simulink model "InvPendIdent"  (Simulink 8.6)
settings: Solver=ode1  SolverMode=SingleTasking  StartTime=0.0  StopTime=40  FixedStep=0.001  RelTol=1e-3
undefined symbols (not defined in the file): Advantech, magnitude, PCI
libraries: sldrtlib x11, simulink x6
settings Model: Creator=Administrator  LastModifiedBy=demo  SimulationMode=external  ExtModeTrigMode=oneshot  ExtModeTrigDuration=100000
settings DataIOCC: LimitDataPoints=off  SignalLoggingName=sigsOut
settings OptimizationCC: BlockReduction=off  BooleanDataType=off  InitFltsAndDblsToZero=on
settings DebuggingCC: SaveWithParameterizedLinksMsg=none  SignalResolutionControl=TryResolveAllWithWarning  SolverPrmCheckMsg=none  MultiTaskDSMMsg=warning  MultiTaskCondExecSysMsg=none  FcnCallInpInsideContextMsg=UseLocalSettings
settings HardwareCC: ProdBitPerLong=64  ProdBitPerPointer=64  ProdIntDivRoundTo=Zero  ProdEndianess=LittleEndian  ProdWordSize=64  ProdHWDeviceType=Intel->x86-64  TargetBitPerLong=64  TargetBitPerPointer=64  TargetIntDivRoundTo=Zero  TargetEndianess=LittleEndian  TargetWordSize=64  TargetHWDeviceType=Intel->x86-64
settings RTWCC: SystemTargetFile=sldrt.tlc  TemplateMakefile=sldrt.tmf  Description=Simulink Desktop Real-Time  RTWCompilerOptimization=on
settings CodeAppCC: MaxIdLength=95
settings SimulinkDesktopRealTimeCC: TargetPreCompLibLocation=C:\Program Files\MATLAB\R2015b\toolbox\sldrt\lib\win64  TargetLangStandard=C89/C90 (ANSI)  SupportVariableSizeSignals=off

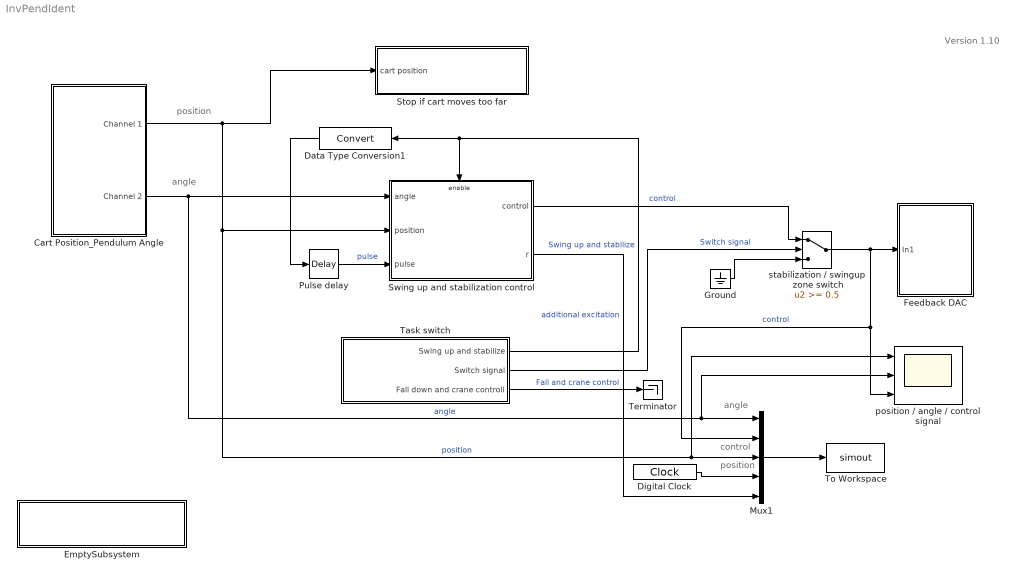
== system InvPendIdent ==
  note: position
  note: angle
  note: Version 1.10
  note: angle
  note: position
  note: control
  Cart Position_Pendulum Angle : Subsystem  mask(Feedback Encoder Block){st=0.001, of1=0, of2=-1024}
      mask prompts: st "Sample Time"; of1 "Channel 1 Offset"; of2 "Channel 2 Offset"
      mask help: Special block to use with the Feedback experiments to read encoder channels using the digital I/O lines
      mask Display:
      | image(imread('bckg.bmp'))
      | disp('PCI1711 \n Lab I/O Board \n\n\n Feedback Encoder')
  Data Type Conversion1 : DataTypeConversion
  Digital Clock : DigitalClock  SampleTime=0.001
  EmptySubsystem : Subsystem
      mask Display:
      | image(imread('FB-inst-blue2.jpg'))
      | disp('\n\nFeedback Instruments Limited')
  Feedback DAC : Subsystem  mask(DAC Unit for Feedback Experiments){st=0.001, ch=1}
      mask prompts: st "Sample Time"; ch "Output Channel"
      mask help:
      | Digital to Analog Output  for Feedback Experiments
      | using Advantech PCI1711  I/O board
      mask Display:
      | image(imread('bckg.bmp'))
      | disp('PCI1711 \n Lab I/O Board \n\n Feedback  DAC')
  Ground : Ground
  Mux1 : Mux  Inputs=5
  Pulse delay : TransportDelay  DelayTime=0.3  FixedBuffer=on
  Stop if cart moves too far : Subsystem
      mask Display:
      | image(imread('bckg.bmp'))
      | disp('Stop if cart moves too far')
  Swing up and stabilization control : Subsystem  TreatAsAtomicUnit=on
      mask Display:
      | image(imread('bckg.bmp'))
      | disp('Swing up \nand stabilization control')
  Task switch : Subsystem
      mask Display:
      | image(imread('bckg.bmp'))
      | disp('Task switch')
  Terminator : Terminator
  To Workspace : ToWorkspace  VariableName=simout  SampleTime=0.001
  position / angle / control signal : Scope  NumInputPorts=3
      mask Display: image(imread('scope.jpg'))
  stabilization / swingup  zone switch : Switch  Threshold=0.5
  wires:
  Cart Position_Pendulum Angle/1(Channel 1) -> Stop if cart moves too far/1(cart position), Swing up and stabilization control/2(position), Mux1/3, position / angle / control signal/1  "position"
  Cart Position_Pendulum Angle/2(Channel 2) -> Swing up and stabilization control/1(angle), Mux1/1, position / angle / control signal/2  "angle"
  stabilization / swingup  zone switch/1 -> Feedback DAC/1(In1), Mux1/2, position / angle / control signal/3  "control"
  Swing up and stabilization control/1(control) -> stabilization / swingup  zone switch/1  "control"
  Pulse delay/1 -> Swing up and stabilization control/3(pulse)  "pulse"
  Data Type Conversion1/1 -> Pulse delay/1
  Task switch/2(Switch signal) -> stabilization / swingup  zone switch/2  "Switch signal"
  Mux1/1 -> To Workspace/1
  Task switch/3(Fall down and crane controll) -> Terminator/1  "Fall and crane control"
  Ground/1 -> stabilization / swingup  zone switch/3
  Task switch/1(Swing up and stabilize) -> Data Type Conversion1/1, Swing up and stabilization control/Enable  "Swing up and stabilize"
  Digital Clock/1 -> Mux1/4
  Swing up and stabilization control/2(r) -> Mux1/5  "additional excitation"

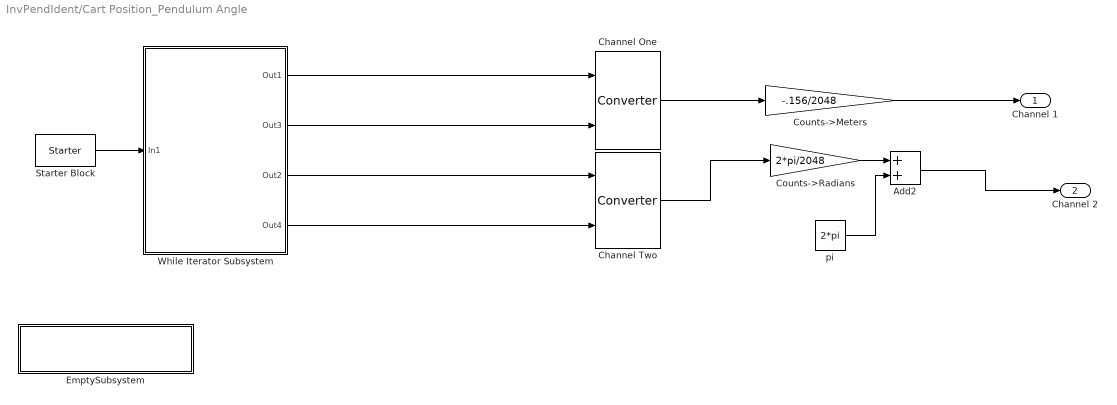
== system InvPendIdent/Cart Position_Pendulum Angle ==
  Add2 : Sum
  Channel One : S-Function  FunctionName=Converter  Parameters=of1,st  SFunctionDeploymentMode=off  EnableBusSupport=off
  Channel Two : S-Function  FunctionName=Converter  Parameters=of2,st  SFunctionDeploymentMode=off  EnableBusSupport=off
  Counts->Meters : Gain  Gain=-.156/2048  SaturateOnIntegerOverflow=on  OutDataTypeStr=Inherit: Same as input  ParamDataTypeStr=Inherit: Same as input
  Counts->Radians : Gain  Gain=2*pi/2048  SaturateOnIntegerOverflow=on  OutDataTypeStr=Inherit: Same as input  ParamDataTypeStr=Inherit: Same as input
  EmptySubsystem : Subsystem
      mask Display:
      | image(imread('FB-inst-blue2.jpg'))
      | disp('\n\nFeedback Instruments Limited')
  Starter Block : S-Function  FunctionName=Starter  Parameters=sample_time  SFunctionDeploymentMode=off  EnableBusSupport=off  mask{sample_time=st}
      mask prompts: sample_time "Sample Time:"
  While Iterator Subsystem : Subsystem  TreatAsAtomicUnit=on
  pi : Constant  Value=2*pi
  Channel 1 : Outport
  Channel 2 : Outport  Port=2
  wires:
  Add2/1 -> Channel 2/1
  Channel Two/1 -> Counts->Radians/1
  pi/1 -> Add2/2
  Counts->Radians/1 -> Add2/1
  Counts->Meters/1 -> Channel 1/1
  Starter Block/1 -> While Iterator Subsystem/1(In1)
  While Iterator Subsystem/1(Out1) -> Channel One/1
  While Iterator Subsystem/2(Out3) -> Channel One/2
  While Iterator Subsystem/3(Out2) -> Channel Two/1
  While Iterator Subsystem/4(Out4) -> Channel Two/2
  Channel One/1 -> Counts->Meters/1

== system InvPendIdent/EmptySubsystem ==

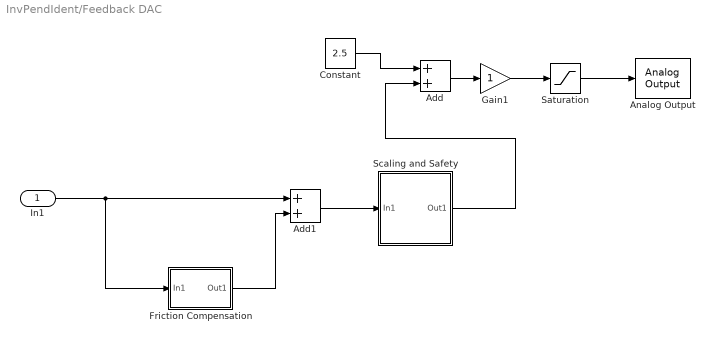
== system InvPendIdent/Feedback DAC ==
  In1 : Inport
  Add : Sum  OutDataTypeStr=Inherit: Same as first input
  Add1 : Sum
  Analog Output : sldrtlib/Analog Output  SampleTime=st  MaxMissedTicks=10  ShowMissedTicks=off  YieldWhenWaiting=off  DrvName=Advantech/PCI-1711  DrvAddress=4294967295  DrvOptions=zeros(1,0)  Channels=ch  RangeMode=1  VoltRange=2  InitialValue=2.5  FinalValue=2.5
      settings: AttributesFormatString=Advantech\nPCI-1711 [auto]
  Constant : Constant  Value=2.5
  Friction Compensation : Subsystem  mask(linear){frictionCompNeg=.1, frictionCompPos=.1}
      mask prompts: frictionCompNeg "Friction Compensation Magnitude in Negative Direction"; frictionCompPos "Friction Compensation Magnitude in Positive Direction"
      mask Display: plot(0,0,100,100,[40,30,20],[87,85,80],[46,54,54,46,46],[90,90,80,80,90],[46,45,45,46,54,55,55,54,46],[78,80,90,91,91,90,80,78,78],[51,51,49,49],[78,10,10,78],[90,80,70,60],[70,80,85,88],[20,10],[80,70],[20,20,15],[73,80,80],[85,80,80],[80,80,74])
  Gain1 : Gain
  Saturation : Saturate  UpperLimit=5.0  LowerLimit=0
  Scaling and Safety : Subsystem
  wires:
  Add1/1 -> Scaling and Safety/1(In1)
  In1/1 -> Add1/1, Friction Compensation/1(In1)
  Friction Compensation/1(Out1) -> Add1/2
  Constant/1 -> Add/1
  Saturation/1 -> Analog Output/1
  Add/1 -> Gain1/1
  Gain1/1 -> Saturation/1
  Scaling and Safety/1(Out1) -> Add/2

== system InvPendIdent/Stop if cart moves too far ==
  cart position : Inport
  Abs3 : Abs
  Compare To Constant1 : simulink/Logic and Bit Operations/Compare To Constant  relop=>  const=0.4  OutDataTypeStr=boolean  ZeroCross=off
  Data Type Conversion1 : DataTypeConversion
  Stop Simulation if cart moves to far : Stop
  wires:
  Abs3/1 -> Compare To Constant1/1
  Compare To Constant1/1 -> Data Type Conversion1/1
  Data Type Conversion1/1 -> Stop Simulation if cart moves to far/1
  cart position/1 -> Abs3/1

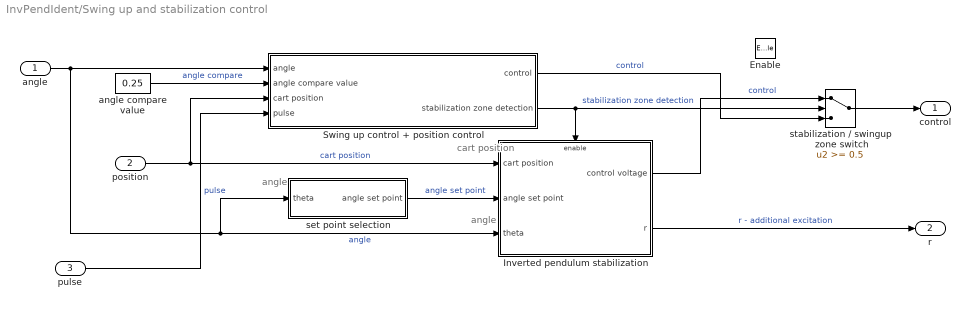
== system InvPendIdent/Swing up and stabilization control ==
  note: angle
  note: cart position
  note: angle
  angle : Inport
  position : Inport  Port=2
  pulse : Inport  Port=3
  Enable : EnablePort
  Inverted pendulum stabilization : Subsystem  TreatAsAtomicUnit=on
      mask Display:
      | image(imread('bckg.bmp'))
      | disp('Inverted pendulum \nstabilization')
  Swing up control + position control : Subsystem
      mask Display:
      | image(imread('bckg.bmp'))
      | disp('Swing up control \nand position control')
  angle compare value : Constant  Value=0.25
  set point selection : Subsystem
      mask Display:
      | image(imread('bckg.bmp'))
      | disp('set point selection')
  stabilization / swingup  zone switch : Switch  Threshold=0.5
  control : Outport
  r : Outport  Port=2
  wires:
  angle/1 -> Swing up control + position control/1(angle), set point selection/1(theta), Inverted pendulum stabilization/3(theta)  "angle"
  Swing up control + position control/1(control) -> stabilization / swingup  zone switch/3  "control"
  Inverted pendulum stabilization/1(control voltage) -> stabilization / swingup  zone switch/1  "control"
  set point selection/1(angle set point) -> Inverted pendulum stabilization/2(angle set point)  "angle set point"
  Swing up control + position control/2(stabilization zone detection) -> stabilization / swingup  zone switch/2, Inverted pendulum stabilization/Enable  "stabilization zone detection"
  angle compare value/1 -> Swing up control + position control/2(angle compare value)  "angle compare"
  position/1 -> Inverted pendulum stabilization/1(cart position), Swing up control + position control/3(cart position)  "cart position"
  stabilization / swingup  zone switch/1 -> control/1
  pulse/1 -> Swing up control + position control/4(pulse)  "pulse"
  Inverted pendulum stabilization/2(r) -> r/1  "r - additional excitation"

== system InvPendIdent/Task switch ==
  Compare To Constant : simulink/Logic and Bit Operations/Compare To Constant  relop=<  const=0.5  OutDataTypeStr=boolean  ZeroCross=off
  Compare To Constant1 : simulink/Logic and Bit Operations/Compare To Constant  relop=>  const=0.5  OutDataTypeStr=boolean  ZeroCross=off
  Pulse Generator : DiscretePulseGenerator  PulseType=Time based  Period=60  PulseWidth=90
  Swing up and stabilize : Outport
  Switch signal : Outport  Port=2
  Fall down and crane controll : Outport  Port=3
  wires:
  Pulse Generator/1 -> Compare To Constant1/1, Switch signal/1, Compare To Constant/1
  Compare To Constant1/1 -> Swing up and stabilize/1
  Compare To Constant/1 -> Fall down and crane controll/1

== system InvPendIdent/Cart Position_Pendulum Angle/EmptySubsystem ==

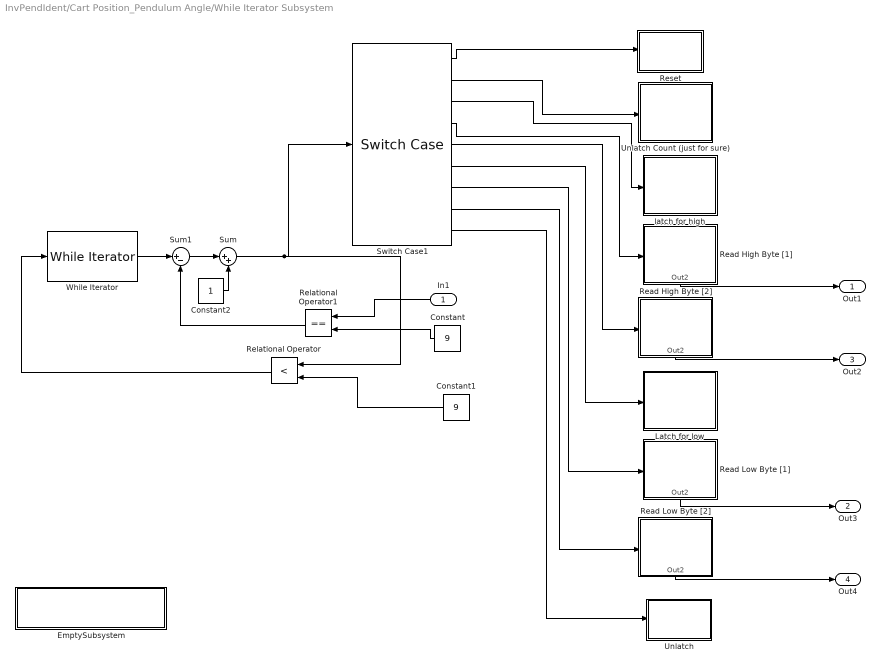
== system InvPendIdent/Cart Position_Pendulum Angle/While Iterator Subsystem ==
  In1 : Inport
  Constant : Constant  Value=9
  Constant1 : Constant  Value=9
  Constant2 : Constant
  EmptySubsystem : Subsystem
      mask Display:
      | image(imread('FB-inst-blue2.jpg'))
      | disp('\n\nFeedback Instruments Limited')
  Latch for low : Subsystem  TreatAsAtomicUnit=on
  Read High Byte [1] : Subsystem  TreatAsAtomicUnit=on
  Read High Byte [2] : Subsystem  TreatAsAtomicUnit=on
  Read Low Byte [1] : Subsystem  TreatAsAtomicUnit=on
  Read Low Byte [2] : Subsystem  TreatAsAtomicUnit=on
  Relational Operator : RelationalOperator  Operator=<  OutDataTypeStr=boolean
  Relational Operator1 : RelationalOperator  Operator===  OutDataTypeStr=boolean
  Reset : Subsystem  TreatAsAtomicUnit=on
  Sum : Sum  Inputs=|++
  Sum1 : Sum  Inputs=|+-  OutDataTypeStr=Inherit: Same as first input
  Switch Case1 : SwitchCase  CaseConditions={1,2,3,4,5,6,7,8,9}  ShowDefaultCase=off
  Unlatch : Subsystem  TreatAsAtomicUnit=on
  "Unlatch Count (just for sure) " : Subsystem  TreatAsAtomicUnit=on
  While Iterator : WhileIterator  MaxIters=9  WhileBlockType=do-while  ResetStates=reset  ShowIterationPort=on  OutputDataType=int8
  latch for high : Subsystem  TreatAsAtomicUnit=on
  Out1 : Outport
  Out3 : Outport  Port=2
  Out2 : Outport  Port=3
  Out4 : Outport  Port=4
  wires:
  Relational Operator/1 -> While Iterator/1
  In1/1 -> Relational Operator1/1
  Constant/1 -> Relational Operator1/2
  Relational Operator1/1 -> Sum1/2
  While Iterator/1 -> Sum1/1
  Switch Case1/1 -> Reset/Action
  Switch Case1/2 -> "Unlatch Count (just for sure) "/Action
  Constant1/1 -> Relational Operator/2
  Read High Byte [1]/1(Out2) -> Out1/1
  Read High Byte [2]/1(Out2) -> Out2/1
  Read Low Byte [1]/1(Out2) -> Out3/1
  Read Low Byte [2]/1(Out2) -> Out4/1
  Sum1/1 -> Sum/1
  Sum/1 -> Switch Case1/1, Relational Operator/1
  Constant2/1 -> Sum/2
  Switch Case1/3 -> latch for high/Action
  Switch Case1/4 -> Read High Byte [1]/Action
  Switch Case1/5 -> Read High Byte [2]/Action
  Switch Case1/6 -> Latch for low/Action
  Switch Case1/7 -> Read Low Byte [1]/Action
  Switch Case1/8 -> Read Low Byte [2]/Action
  Switch Case1/9 -> Unlatch/Action

== system InvPendIdent/Feedback DAC/Friction Compensation ==
  In1 : Inport
  " " : Gain  Gain=frictionCompPos  SaturateOnIntegerOverflow=on  OutDataTypeStr=Inherit: Same as input  ParamDataTypeStr=Inherit: Same as input
  3 : Switch  SaturateOnIntegerOverflow=on  InputSameDT=on
  Gain3 : Gain  Gain=frictionCompNeg  SaturateOnIntegerOverflow=on  OutDataTypeStr=Inherit: Same as input  ParamDataTypeStr=Inherit: Same as input
  Sign2 : Signum  Tag=T
  Out1 : Outport  InitialOutput=0
  wires:
  3/1 -> Out1/1
  Sign2/1 -> 3/2, " "/1, Gain3/1
  Gain3/1 -> 3/3
  " "/1 -> 3/1
  In1/1 -> Sign2/1

== system InvPendIdent/Feedback DAC/Scaling and Safety ==
  In1 : Inport
  -1 : Gain  Gain=-1  SaturateOnIntegerOverflow=on  OutDataTypeStr=Inherit: Same as input  ParamDataTypeStr=Inherit: Same as input
  Saturation : Saturate  UpperLimit=2.5  LowerLimit=-2.5
  Out1 : Outport
  wires:
  -1/1 -> Saturation/1  "actual LoadPosition"
  In1/1 -> -1/1
  Saturation/1 -> Out1/1

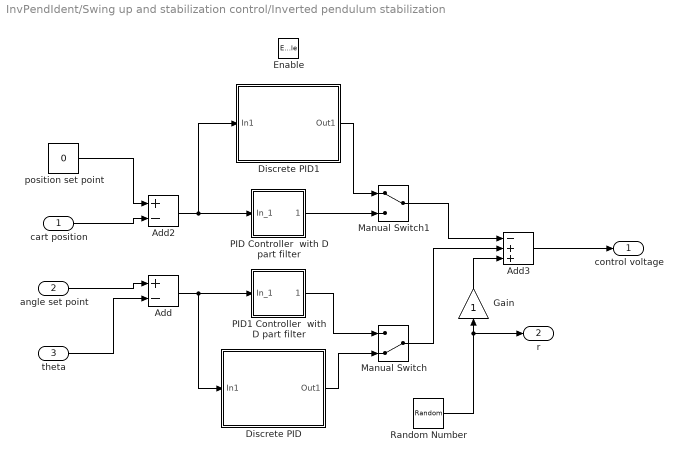
== system InvPendIdent/Swing up and stabilization control/Inverted pendulum stabilization ==
  cart position : Inport
  angle set point : Inport  Port=2
  theta : Inport  Port=3
  Enable : EnablePort
  Add : Sum  Inputs=+-
  Add2 : Sum  Inputs=+-
  Add3 : Sum  Inputs=-++
  Discrete PID : Subsystem  mask{Kp=20, Ki=0.1, Kd=2}
      mask Display:
      | image(imread('bckg.bmp'))
      | disp('PID')
  Discrete PID1 : Subsystem  mask{Kp=7, Ki=0.1, Kd=2}
      mask Display:
      | image(imread('bckg.bmp'))
      | disp('PID')
  Gain : Gain
  Manual Switch : ManualSwitch  CurrentSetting=0
  Manual Switch1 : ManualSwitch
  PID Controller  with D part filter : Subsystem  AncestorBlock=simulink_extras/Additional Linear/PID Controller  mask(PID Controller){P=7, I=0.1, D=2}
      mask prompts: P "Proportional:"; I "Integral:"; D "Derivative:"
      mask help:
      | Enter expressions for proportional, integral, and derivative terms.
      | P+I/s+Ds
      mask Help: This block implements a PID controller where parameters are entered for the Proportional, Integral and Derivative terms. Unmask this block to see how it works. The derivative term is implemented using a true derivative block.
      mask Display:
      | image(imread('bckg.bmp'))
      | disp('PID')
  PID1 Controller  with D part filter : Subsystem  AncestorBlock=simulink_extras/Additional Linear/PID Controller  mask(PID Controller){P=20, I=0.1, D=2}
      mask prompts: P "Proportional:"; I "Integral:"; D "Derivative:"
      mask help:
      | Enter expressions for proportional, integral, and derivative terms.
      | P+I/s+Ds
      mask Help: This block implements a PID controller where parameters are entered for the Proportional, Integral and Derivative terms. Unmask this block to see how it works. The derivative term is implemented using a true derivative block.
      mask Display:
      | image(imread('bckg.bmp'))
      | disp('PID')
  Random Number : RandomNumber  Variance=0.3  Seed=425745685  SampleTime=0.05
  position set point : Constant  Value=0
  control voltage : Outport
  r : Outport  Port=2
  wires:
  Add/1 -> PID1 Controller  with D part filter/1(In_1), Discrete PID/1(In1)
  position set point/1 -> Add2/1
  Add2/1 -> PID Controller  with D part filter/1(In_1), Discrete PID1/1(In1)
  cart position/1 -> Add2/2
  theta/1 -> Add/2
  angle set point/1 -> Add/1
  Add3/1 -> control voltage/1
  Random Number/1 -> r/1, Gain/1
  Manual Switch/1 -> Add3/2
  PID1 Controller  with D part filter/1(Out_1) -> Manual Switch/1
  Discrete PID/1(Out1) -> Manual Switch/2
  Gain/1 -> Add3/3
  PID Controller  with D part filter/1(Out_1) -> Manual Switch1/2
  Manual Switch1/1 -> Add3/1
  Discrete PID1/1(Out1) -> Manual Switch1/1

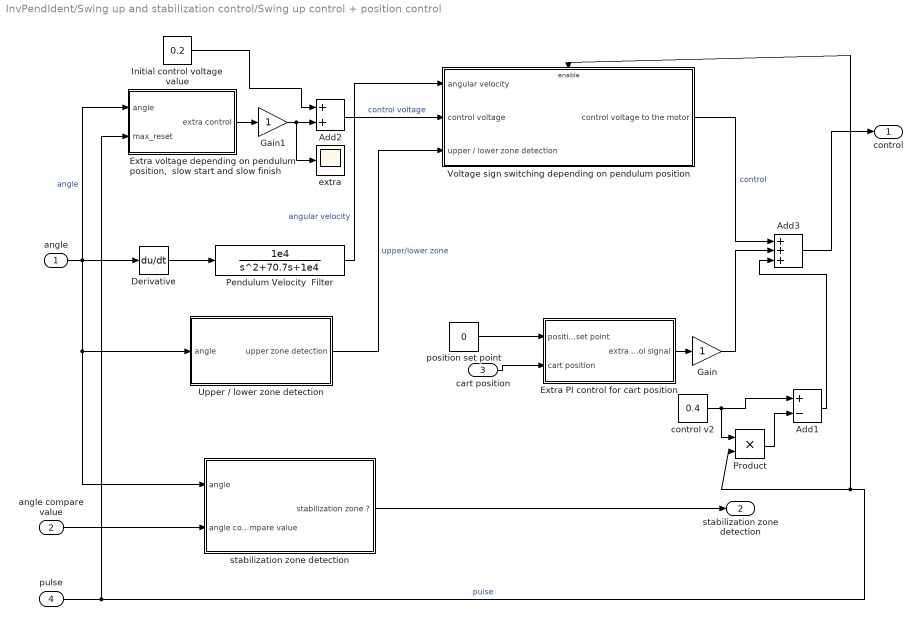
== system InvPendIdent/Swing up and stabilization control/Swing up control + position control ==
  angle : Inport
  angle compare value : Inport  Port=2
  cart position : Inport  Port=3
  pulse : Inport  Port=4
  Add1 : Sum  Inputs=+-
  Add2 : Sum
  Add3 : Sum  Inputs=+++
  Derivative : Derivative
  Extra PI control for cart position : Subsystem
  "Extra voltage depending on pendulum position,  slow start and slow finish" : Subsystem
      mask Display:
      | image(imread('bckg.bmp'))
      | disp('Extra voltage')
  Gain : Gain
  Gain1 : Gain
  Initial control voltage value : Constant  Value=0.2
  Pendulum Velocity  Filter : TransferFcn  Numerator=[1e4]  Denominator=[1 70.7 1e4]
  Product : Product  RndMeth=Zero
  Upper / lower zone detection : Subsystem
      mask Display:
      | image(imread('bckg.bmp'))
      | disp('Upper / lower zone \ndetection')
  Voltage sign switching depending on pendulum position : Subsystem
      mask Display:
      | image(imread('bckg.bmp'))
      | disp('Voltage sign switching depending on \npendulum position')
  control v2 : Constant  Value=0.4
  extra : Scope
      mask Display: image(imread('scope.jpg'))
  position set point : Constant  Value=0
  "stabilization zone detection " : Subsystem
      mask Display:
      | image(imread('bckg.bmp'))
      | disp('stabilization zone detection')
  control : Outport
  stabilization zone detection : Outport  Port=2
  wires:
  Upper / lower zone detection/1(upper zone detection) -> Voltage sign switching depending on pendulum position/3(upper / lower zone detection)  "upper/lower zone"
  Initial control voltage value/1 -> Add2/1
  Add2/1 -> Voltage sign switching depending on pendulum position/2(control voltage)  "control voltage"
  angle/1 -> "Extra voltage depending on pendulum position,  slow start and slow finish"/1(angle), Derivative/1, Upper / lower zone detection/1(angle), "stabilization zone detection "/1(angle)  "angle"
  Derivative/1 -> Pendulum Velocity  Filter/1
  Pendulum Velocity  Filter/1 -> Voltage sign switching depending on pendulum position/1(angular velocity)  "angular velocity"
  "stabilization zone detection "/1(stabilization zone ?) -> stabilization zone detection/1
  angle compare value/1 -> "stabilization zone detection "/2(angle compare value)
  position set point/1 -> Extra PI control for cart position/1(position set point)
  cart position/1 -> Extra PI control for cart position/2(cart position)
  Extra PI control for cart position/1(extra control signal) -> Gain/1
  Voltage sign switching depending on pendulum position/1(control voltage to the motor) -> Add3/1  "control"
  Add3/1 -> control/1
  Gain/1 -> Add3/2
  "Extra voltage depending on pendulum position,  slow start and slow finish"/1(extra control) -> Gain1/1
  Gain1/1 -> Add2/2, extra/1
  pulse/1 -> Product/2, Voltage sign switching depending on pendulum position/Enable, "Extra voltage depending on pendulum position,  slow start and slow finish"/2(max_reset)  "pulse"
  Add1/1 -> Add3/3
  control v2/1 -> Add1/1, Product/1
  Product/1 -> Add1/2

== system InvPendIdent/Swing up and stabilization control/set point selection ==
  theta : Inport
  0 : Constant  Value=0
  2*pi : Constant  Value=2*pi
  Abs : Abs
  zero velocity : Switch  Threshold=pi
  angle set point : Outport
  wires:
  zero velocity/1 -> angle set point/1
  theta/1 -> Abs/1
  Abs/1 -> zero velocity/2
  2*pi/1 -> zero velocity/1
  0/1 -> zero velocity/3

== system InvPendIdent/Cart Position_Pendulum Angle/While Iterator Subsystem/EmptySubsystem ==

== system InvPendIdent/Cart Position_Pendulum Angle/While Iterator Subsystem/Latch for low ==
  Action Port : ActionPort  ActionType=case
  Constant : Constant  Value=6  OutDataTypeStr=double
  Digital Output : sldrtlib/Digital Output  SampleTime=-1  MaxMissedTicks=10  ShowMissedTicks=off  YieldWhenWaiting=off  DrvName=Advantech/PCI-1711  DrvAddress=4294967295  DrvOptions=zeros(1,0)  Channels=1  BitMode=2  InitialValue=0  FinalValue=0
      settings: AttributesFormatString=Advantech\nPCI-1711 [auto]
  wires:
  Constant/1 -> Digital Output/1

== system InvPendIdent/Cart Position_Pendulum Angle/While Iterator Subsystem/Read High Byte [1] ==
  Action Port : ActionPort  ActionType=case
  Constant1 : Constant  Value=[1 2 4 8 16 32 64 128]
  Digital Input1 : sldrtlib/Digital Input  SampleTime=-1  MaxMissedTicks=10  ShowMissedTicks=off  YieldWhenWaiting=off  DrvName=Advantech/PCI-1711  DrvAddress=4294967295  DrvOptions=zeros(1,0)  Channels=[1,2,3,4,5,6,7,8]  BitMode=1  DataType=1
      settings: AttributesFormatString=Advantech\nPCI-1711 [auto]
  Dot Product : DotProduct  InputSameDT=on  OutDataTypeStr=Inherit: Inherit via internal rule
  Out2 : Outport
  wires:
  Dot Product/1 -> Out2/1
  Constant1/1 -> Dot Product/2
  Digital Input1/1 -> Dot Product/1

== system InvPendIdent/Cart Position_Pendulum Angle/While Iterator Subsystem/Read High Byte [2] ==
  Action Port : ActionPort  ActionType=case
  Constant1 : Constant  Value=[1 2 4 8 16 32 64 128]
  Digital Input1 : sldrtlib/Digital Input  SampleTime=-1  MaxMissedTicks=10  ShowMissedTicks=off  YieldWhenWaiting=off  DrvName=Advantech/PCI-1711  DrvAddress=4294967295  DrvOptions=zeros(1,0)  Channels=[9:16]  BitMode=1  DataType=1
      settings: AttributesFormatString=Advantech\nPCI-1711 [auto]
  Dot Product : DotProduct  InputSameDT=on  OutDataTypeStr=Inherit: Inherit via internal rule
  Out2 : Outport
  wires:
  Digital Input1/1 -> Dot Product/1
  Constant1/1 -> Dot Product/2
  Dot Product/1 -> Out2/1

== system InvPendIdent/Cart Position_Pendulum Angle/While Iterator Subsystem/Read Low Byte [1] ==
  Action Port : ActionPort  ActionType=case
  Constant1 : Constant  Value=[1 2 4 8 16 32 64 128]
  Digital Input1 : sldrtlib/Digital Input  SampleTime=-1  MaxMissedTicks=10  ShowMissedTicks=off  YieldWhenWaiting=off  DrvName=Advantech/PCI-1711  DrvAddress=4294967295  DrvOptions=zeros(1,0)  Channels=[1:8]  BitMode=1  DataType=1
      settings: AttributesFormatString=Advantech\nPCI-1711 [auto]
  Dot Product : DotProduct  InputSameDT=on  OutDataTypeStr=Inherit: Inherit via internal rule
  Out2 : Outport
  wires:
  Digital Input1/1 -> Dot Product/1
  Constant1/1 -> Dot Product/2
  Dot Product/1 -> Out2/1

== system InvPendIdent/Cart Position_Pendulum Angle/While Iterator Subsystem/Read Low Byte [2] ==
  Action Port : ActionPort  ActionType=case
  Constant1 : Constant  Value=[1 2 4 8 16 32 64 128]
  Digital Input1 : sldrtlib/Digital Input  SampleTime=-1  MaxMissedTicks=10  ShowMissedTicks=off  YieldWhenWaiting=off  DrvName=Advantech/PCI-1711  DrvAddress=4294967295  DrvOptions=zeros(1,0)  Channels=[9:16]  BitMode=1  DataType=1
      settings: AttributesFormatString=Advantech\nPCI-1711 [auto]
  Dot Product : DotProduct  InputSameDT=on  OutDataTypeStr=Inherit: Inherit via internal rule
  Out2 : Outport
  wires:
  Constant1/1 -> Dot Product/2
  Digital Input1/1 -> Dot Product/1
  Dot Product/1 -> Out2/1

== system InvPendIdent/Cart Position_Pendulum Angle/While Iterator Subsystem/Reset ==
  Action Port : ActionPort  ActionType=case
  Constant : Constant  Value=3  OutDataTypeStr=double
  Digital Output1 : sldrtlib/Digital Output  SampleTime=-1  MaxMissedTicks=10  ShowMissedTicks=off  YieldWhenWaiting=off  DrvName=Advantech/PCI-1711  DrvAddress=4294967295  DrvOptions=zeros(1,0)  Channels=1  BitMode=2  InitialValue=0  FinalValue=0
      settings: AttributesFormatString=Advantech\nPCI-1711 [auto]
  Subsystem : Subsystem
  wires:
  Constant/1 -> Subsystem/1(In1)
  Subsystem/1(Out1) -> Digital Output1/1

== system InvPendIdent/Cart Position_Pendulum Angle/While Iterator Subsystem/Unlatch ==
  Action Port : ActionPort  ActionType=case
  Constant : Constant  Value=7  OutDataTypeStr=double
  Digital Output1 : sldrtlib/Digital Output  SampleTime=-1  MaxMissedTicks=10  ShowMissedTicks=off  YieldWhenWaiting=off  DrvName=Advantech/PCI-1711  DrvAddress=4294967295  DrvOptions=zeros(1,0)  Channels=1  BitMode=2  InitialValue=0  FinalValue=0
      settings: AttributesFormatString=Advantech\nPCI-1711 [auto]
  wires:
  Constant/1 -> Digital Output1/1

== system InvPendIdent/Cart Position_Pendulum Angle/While Iterator Subsystem/Unlatch Count (just for sure)  ==
  Action Port : ActionPort  ActionType=case
  Constant : Constant  Value=7  OutDataTypeStr=double
  Digital Output : sldrtlib/Digital Output  SampleTime=-1  MaxMissedTicks=10  ShowMissedTicks=off  YieldWhenWaiting=off  DrvName=Advantech/PCI-1711  DrvAddress=4294967295  DrvOptions=zeros(1,0)  Channels=1  BitMode=2  InitialValue=0  FinalValue=0
      settings: AttributesFormatString=Advantech\nPCI-1711 [auto]
  wires:
  Constant/1 -> Digital Output/1

== system InvPendIdent/Cart Position_Pendulum Angle/While Iterator Subsystem/latch for high ==
  Action Port : ActionPort  ActionType=case
  Constant : Constant  Value=4  OutDataTypeStr=double
  Digital Output : sldrtlib/Digital Output  SampleTime=-1  MaxMissedTicks=10  ShowMissedTicks=off  YieldWhenWaiting=off  DrvName=Advantech/PCI-1711  DrvAddress=4294967295  DrvOptions=zeros(1,0)  Channels=1  BitMode=2  InitialValue=0  FinalValue=0
      settings: AttributesFormatString=Advantech\nPCI-1711 [auto]
  wires:
  Constant/1 -> Digital Output/1

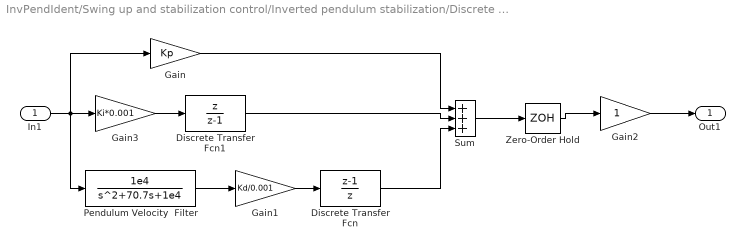
== system InvPendIdent/Swing up and stabilization control/Inverted pendulum stabilization/Discrete PID ==
  In1 : Inport
  Discrete Transfer Fcn : DiscreteTransferFcn  Numerator=[1 -1]  Denominator=[1 0]  SampleTime=0.001
  Discrete Transfer Fcn1 : DiscreteTransferFcn  Numerator=[1 0]  Denominator=[1 -1]  SampleTime=0.001
  Gain : Gain  Gain=Kp  SampleTime=0.001
  Gain1 : Gain  Gain=Kd/0.001  SampleTime=0.001
  Gain2 : Gain  SampleTime=0.001
  Gain3 : Gain  Gain=Ki*0.001  SampleTime=0.001
  Pendulum Velocity  Filter : TransferFcn  Numerator=[1e4]  Denominator=[1 70.7 1e4]
  Sum : Sum  Inputs=+++  SampleTime=0.01
  Zero-Order Hold : ZeroOrderHold  SampleTime=0.001
  Out1 : Outport
  wires:
  Zero-Order Hold/1 -> Gain2/1
  Gain2/1 -> Out1/1
  Sum/1 -> Zero-Order Hold/1
  Gain3/1 -> Discrete Transfer Fcn1/1
  Discrete Transfer Fcn1/1 -> Sum/2
  Discrete Transfer Fcn/1 -> Sum/3
  Gain1/1 -> Discrete Transfer Fcn/1
  Gain/1 -> Sum/1
  In1/1 -> Gain/1, Gain3/1, Pendulum Velocity  Filter/1
  Pendulum Velocity  Filter/1 -> Gain1/1

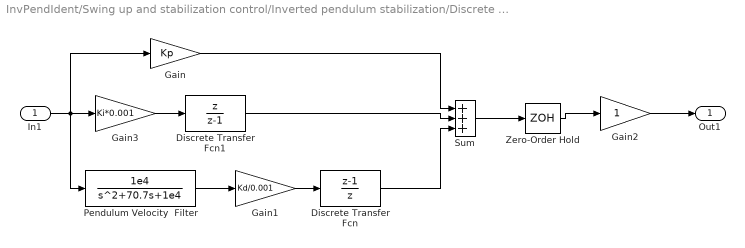
== system InvPendIdent/Swing up and stabilization control/Inverted pendulum stabilization/Discrete PID1 ==
  In1 : Inport
  Discrete Transfer Fcn : DiscreteTransferFcn  Numerator=[1 -1]  Denominator=[1 0]  SampleTime=0.001
  Discrete Transfer Fcn1 : DiscreteTransferFcn  Numerator=[1 0]  Denominator=[1 -1]  SampleTime=0.001
  Gain : Gain  Gain=Kp  SampleTime=0.001
  Gain1 : Gain  Gain=Kd/0.001  SampleTime=0.001
  Gain2 : Gain  SampleTime=0.001
  Gain3 : Gain  Gain=Ki*0.001  SampleTime=0.001
  Pendulum Velocity  Filter : TransferFcn  Numerator=[1e4]  Denominator=[1 70.7 1e4]
  Sum : Sum  Inputs=+++  SampleTime=0.01
  Zero-Order Hold : ZeroOrderHold  SampleTime=0.001
  Out1 : Outport
  wires:
  Pendulum Velocity  Filter/1 -> Gain1/1
  In1/1 -> Pendulum Velocity  Filter/1, Gain3/1, Gain/1
  Gain/1 -> Sum/1
  Gain1/1 -> Discrete Transfer Fcn/1
  Discrete Transfer Fcn/1 -> Sum/3
  Discrete Transfer Fcn1/1 -> Sum/2
  Gain3/1 -> Discrete Transfer Fcn1/1
  Sum/1 -> Zero-Order Hold/1
  Gain2/1 -> Out1/1
  Zero-Order Hold/1 -> Gain2/1

== system InvPendIdent/Swing up and stabilization control/Inverted pendulum stabilization/PID Controller  with D part filter ==
  In_1 : Inport
  D : Gain  Gain=D  SaturateOnIntegerOverflow=on  OutDataTypeStr=Inherit: Same as input  ParamDataTypeStr=Inherit: Same as input
  Derivative : Derivative
  Integral : TransferFcn  Numerator=[I]  Denominator=[1 0]
  Pendulum Velocity  Filter : TransferFcn  Numerator=[1e4]  Denominator=[1 70.7 1e4]
  Proportional : Gain  Gain=P  SaturateOnIntegerOverflow=on  OutDataTypeStr=Inherit: Same as input  ParamDataTypeStr=Inherit: Same as input
  Sum : Sum  Inputs=+++  SaturateOnIntegerOverflow=on  InputSameDT=on  OutDataTypeStr=Inherit: Same as first input
  Out_1 : Outport  InitialOutput=0
  wires:
  Pendulum Velocity  Filter/1 -> Sum/3
  D/1 -> Derivative/1
  Sum/1 -> Out_1/1
  In_1/1 -> Proportional/1, Integral/1, D/1
  Derivative/1 -> Pendulum Velocity  Filter/1
  Integral/1 -> Sum/2
  Proportional/1 -> Sum/1

== system InvPendIdent/Swing up and stabilization control/Inverted pendulum stabilization/PID1 Controller  with D part filter ==
  In_1 : Inport
  D : Gain  Gain=D  SaturateOnIntegerOverflow=on  OutDataTypeStr=Inherit: Same as input  ParamDataTypeStr=Inherit: Same as input
  Derivative : Derivative
  Integral : TransferFcn  Numerator=[I]  Denominator=[1 0]
  Pendulum Velocity  Filter : TransferFcn  Numerator=[1e4]  Denominator=[1 70.7 1e4]
  Proportional : Gain  Gain=P  SaturateOnIntegerOverflow=on  OutDataTypeStr=Inherit: Same as input  ParamDataTypeStr=Inherit: Same as input
  Sum : Sum  Inputs=+++  SaturateOnIntegerOverflow=on  InputSameDT=on  OutDataTypeStr=Inherit: Same as first input
  Out_1 : Outport  InitialOutput=0
  wires:
  Proportional/1 -> Sum/1
  Integral/1 -> Sum/2
  Derivative/1 -> Pendulum Velocity  Filter/1
  In_1/1 -> Integral/1, Proportional/1, D/1
  Sum/1 -> Out_1/1
  D/1 -> Derivative/1
  Pendulum Velocity  Filter/1 -> Sum/3

== system InvPendIdent/Swing up and stabilization control/Swing up control + position control/Extra PI control for cart position ==
  position set point : Inport
  cart position : Inport  Port=2
  Add1 : Sum  Inputs=+-
  PID Controller  with D part filter : Subsystem  AncestorBlock=simulink_extras/Additional Linear/PID Controller  mask(PID Controller){P=0.5, I=0.2, D=0}
      mask prompts: P "Proportional:"; I "Integral:"; D "Derivative:"
      mask help:
      | Enter expressions for proportional, integral, and derivative terms.
      | P+I/s+Ds
      mask Help: This block implements a PID controller where parameters are entered for the Proportional, Integral and Derivative terms. Unmask this block to see how it works. The derivative term is implemented using a true derivative block.
      mask Display:
      | image(imread('bckg.bmp'))
      | disp('PID')
  extra control signal : Outport
  wires:
  Add1/1 -> PID Controller  with D part filter/1(In_1)
  position set point/1 -> Add1/1
  PID Controller  with D part filter/1(Out_1) -> extra control signal/1
  cart position/1 -> Add1/2

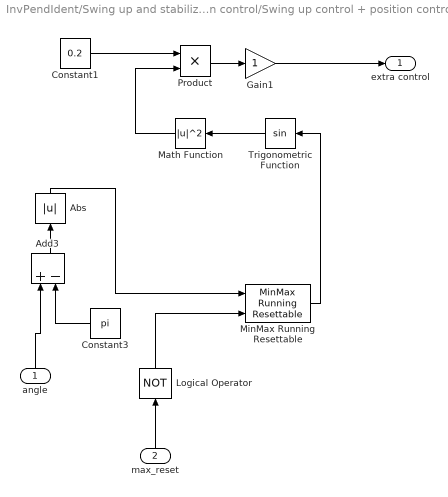
== system InvPendIdent/Swing up and stabilization control/Swing up control + position control/Extra voltage depending on pendulum position,  slow start and slow finish ==
  angle : Inport
  max_reset : Inport  Port=2
  Abs : Abs
  Add3 : Sum  Inputs=+-
  Constant1 : Constant  Value=0.2
  Constant3 : Constant  Value=pi
  Gain1 : Gain
  Logical Operator : Logic  Operator=NOT  AllPortsSameDT=off  OutDataTypeStr=boolean
  Math Function : Math  Operator=magnitude^2  SaturateOnIntegerOverflow=on
  MinMax Running Resettable : simulink/Math Operations/MinMax Running Resettable  Function=max  vinit=0.0
  Product : Product  RndMeth=Zero
  Trigonometric Function : Trigonometry
  extra control : Outport
  wires:
  Product/1 -> Gain1/1
  Constant1/1 -> Product/1
  Constant3/1 -> Add3/2
  Add3/1 -> Abs/1
  Abs/1 -> MinMax Running Resettable/1
  Trigonometric Function/1 -> Math Function/1
  Gain1/1 -> extra control/1
  Math Function/1 -> Product/2
  angle/1 -> Add3/1
  max_reset/1 -> Logical Operator/1
  MinMax Running Resettable/1 -> Trigonometric Function/1
  Logical Operator/1 -> MinMax Running Resettable/2

== system InvPendIdent/Swing up and stabilization control/Swing up control + position control/Upper / lower zone detection ==
  angle : Inport
  Compare To Constant : simulink/Logic and Bit Operations/Compare To Constant  relop=<=  const=pi/2  OutDataTypeStr=uint8  ZeroCross=off
  Compare To Constant1 : simulink/Logic and Bit Operations/Compare To Constant  relop=>=  const=pi/2+pi  OutDataTypeStr=uint8  ZeroCross=off
  Logical Operator : Logic  Operator=OR  AllPortsSameDT=off  OutDataTypeStr=boolean
  upper zone detection : Outport
  wires:
  Compare To Constant/1 -> Logical Operator/1
  Compare To Constant1/1 -> Logical Operator/2
  angle/1 -> Compare To Constant/1, Compare To Constant1/1
  Logical Operator/1 -> upper zone detection/1

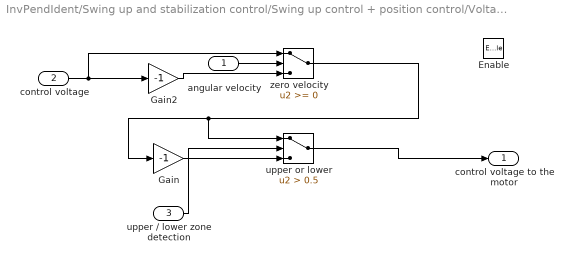
== system InvPendIdent/Swing up and stabilization control/Swing up control + position control/Voltage sign switching depending on pendulum position ==
  angular velocity : Inport
  control voltage : Inport  Port=2
  upper / lower zone detection : Inport  Port=3
  Enable : EnablePort
  Gain : Gain  Gain=-1
  Gain2 : Gain  Gain=-1
  upper or lower : Switch  Criteria=u2 > Threshold  Threshold=0.5
  zero velocity : Switch
  control voltage to the motor : Outport
  wires:
  Gain/1 -> upper or lower/3
  zero velocity/1 -> upper or lower/1, Gain/1
  control voltage/1 -> zero velocity/1, Gain2/1
  Gain2/1 -> zero velocity/3
  angular velocity/1 -> zero velocity/2
  upper or lower/1 -> control voltage to the motor/1
  upper / lower zone detection/1 -> upper or lower/2

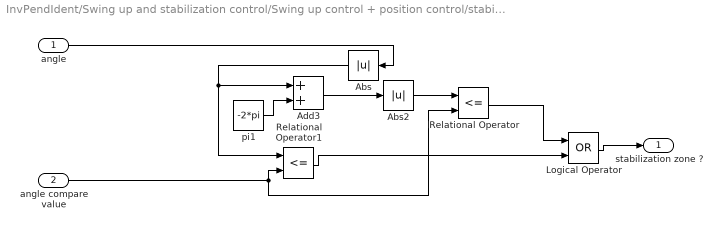
== system InvPendIdent/Swing up and stabilization control/Swing up control + position control/stabilization zone detection  ==
  angle : Inport
  angle compare value : Inport  Port=2
  Abs : Abs
  Abs2 : Abs
  Add3 : Sum
  Logical Operator : Logic  Operator=OR  AllPortsSameDT=off  OutDataTypeStr=boolean
  Relational Operator : RelationalOperator  Operator=<=  OutDataTypeStr=boolean
  Relational Operator1 : RelationalOperator  Operator=<=  OutDataTypeStr=boolean
  pi1 : Constant  Value=-2*pi
  stabilization zone ? : Outport
  wires:
  Abs/1 -> Add3/1, Relational Operator1/1
  Relational Operator1/1 -> Logical Operator/2
  pi1/1 -> Add3/2
  Add3/1 -> Abs2/1
  Relational Operator/1 -> Logical Operator/1
  Abs2/1 -> Relational Operator/1
  angle/1 -> Abs/1
  Logical Operator/1 -> stabilization zone ?/1
  angle compare value/1 -> Relational Operator1/2, Relational Operator/2

== system InvPendIdent/Cart Position_Pendulum Angle/While Iterator Subsystem/Reset/Subsystem ==
  In1 : Inport
  Constant1 : Constant  Value=7  OutDataTypeStr=double
  Digital Output : sldrtlib/Digital Output  SampleTime=-1  MaxMissedTicks=10  ShowMissedTicks=off  YieldWhenWaiting=off  DrvName=Advantech/PCI-1711  DrvAddress=4294967295  DrvOptions=zeros(1,0)  Channels=[1 2 3]  BitMode=2  InitialValue=0  FinalValue=0
      settings: AttributesFormatString=Advantech\nPCI-1711 [auto]
  Out1 : Outport
  wires:
  Constant1/1 -> Out1/1
  In1/1 -> Digital Output/1

== system InvPendIdent/Swing up and stabilization control/Swing up control + position control/Extra PI control for cart position/PID Controller  with D part filter ==
  In_1 : Inport
  D : Gain  Gain=D  SaturateOnIntegerOverflow=on  OutDataTypeStr=Inherit: Same as input  ParamDataTypeStr=Inherit: Same as input
  Derivative : Derivative
  Integral : TransferFcn  Numerator=[I]  Denominator=[1 0]
  Pendulum Velocity  Filter : TransferFcn  Numerator=[1e4]  Denominator=[1 70.7 1e4]
  Proportional : Gain  Gain=P  SaturateOnIntegerOverflow=on  OutDataTypeStr=Inherit: Same as input  ParamDataTypeStr=Inherit: Same as input
  Sum : Sum  Inputs=+++  SaturateOnIntegerOverflow=on  InputSameDT=on  OutDataTypeStr=Inherit: Same as first input
  Out_1 : Outport  InitialOutput=0
  wires:
  Proportional/1 -> Sum/1
  Integral/1 -> Sum/2
  Derivative/1 -> Pendulum Velocity  Filter/1
  In_1/1 -> Integral/1, Proportional/1, D/1
  Sum/1 -> Out_1/1
  D/1 -> Derivative/1
  Pendulum Velocity  Filter/1 -> Sum/3
